simulink model "first_order_tf"  (R2018b)
settings: Solver=ode1  StartTime=0.0  StopTime=10.0  RelTol=1e-3  EnableMultiTasking=on
values from neighbouring files (symbols this model uses):
  den = Simulink.Parameter    [discrete_tf_init.m]    (also in first_order_tf_init.m)
  num = Simulink.Parameter    [discrete_tf_init.m]    (also in first_order_tf_init.m)
settings Model: Creator=C3038028  LastModifiedBy=user
settings DataIOCC: LimitDataPoints=on
settings OptimizationCC: DefaultParameterBehavior=Inlined  LifeSpan=1
settings DebuggingCC: AllowSymbolicDim=off  SFUnexpectedBacktrackingDiag=warning  SFNoUnconditionalDefaultTransitionDiag=warning  SFExecutionAtInitializationDiag=none
settings HardwareCC: TargetBitPerPointer=64  TargetBitPerSizeT=64  TargetBitPerPtrDiffT=64  TargetLongLongMode=on  TargetIntDivRoundTo=Zero  TargetEndianess=LittleEndian  TargetWordSize=64  TargetHWDeviceType=MATLAB Host  ProdEqTarget=off
settings ModelReferenceCC: PropagateSignalLabelsOutOfModel=off
settings SFSimCC: SimUseLocalCustomCode=off  MATLABDynamicMemAlloc=off
settings RTWCC: SystemTargetFile=ert_shrlib.tlc  TemplateMakefile=ert_default_tmf  Description=Embedded Coder (host-based shared library target)  RTWUseLocalCustomCode=off  BuildConfiguration=Faster Runs
settings CodeAppCC: IgnoreCustomStorageClasses=off  StateflowObjectComments=on
settings STFCustomTargetCC: GenerateSampleERTMain=on  ParMdlRefBuildCompliant=on  CompOptLevelCompliant=on  CombineOutputUpdateFcns=on  ERTCustomFileBanners=on  SupportNonInlinedSFcns=off  RemoveResetFunc=on  MATLABClassNameForMDSCustomization=Simulink.SoftwareTarget.ERTCustomization  ModelStepFunctionPrototypeControlCompliant=on  UseToolchainInfoCompliant=on  SystemTargetFile=ert_shrlib.tlc
settings ERTTargetCC: MultiwordLength=2048  GenerateSampleERTMain=on  ConcurrentExecutionCompliant=off  SupportContinuousTime=on  CPPClassGenCompliant=off  InlinedParameterPlacement=NonHierarchical  ERTCustomFileTemplate=example_file_process.tlc  ConvertIfToSwitch=off  SuppressUnreachableDefaultCases=off
settings ConfigComp: CovMetricSettings=dw  CovHtmlReporting=on  CovSaveCumulativeToWorkspaceVar=on  CovSaveSingleToWorkspaceVar=on  CovExternalEMLEnable=off

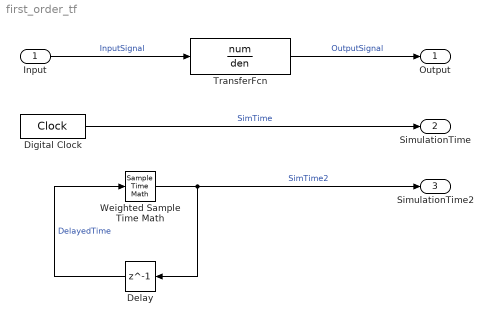
== system first_order_tf ==
  Input : Inport
  Delay : Delay  DelayLength=1
  Digital Clock : DigitalClock  SampleTime=0.01
  TransferFcn : TransferFcn  Numerator=num  Denominator=den
  Weighted Sample Time Math : SampleTimeMath  weightValue=1
  Output : Outport
  SimulationTime : Outport  Port=2
  SimulationTime2 : Outport  Port=3
  wires:
  Input/1 -> TransferFcn/1  "InputSignal"
  TransferFcn/1 -> Output/1  "OutputSignal"
  Digital Clock/1 -> SimulationTime/1  "SimTime"
  Weighted Sample Time Math/1 -> SimulationTime2/1, Delay/1  "SimTime2"
  Delay/1 -> Weighted Sample Time Math/1  "DelayedTime"
